simulink model "Lombardy"  (Simulink 7.9)
settings: Solver=ode45  StartTime=0.0  StopTime=10.0  RelTol=1e-3
undefined symbols (not defined in the file or in its folder): f_NODE01, f_NODE02, f_NODE03, f_NODE04, f_NODE05, f_NODE06, f_NODE07, f_NODE08, f_NODE09, f_NODE10, f_NODE11, f_NODE12, f_NODE13, f_NODE14, f_NODE15, f_NODE16, f_NODE17, f_NODE18, f_NODE19, f_NODE20, f_NODE21, f_NODE22, f_NODE23, f_NODE24, f_NODE25, f_NODE26, f_NODE27, f_NODE28, f_NODE29, f_NODE30, f_NODE31, f_NODE32, r_NODE01, r_NODE02, r_NODE03, r_NODE04, r_NODE05, r_NODE06, r_NODE07, r_NODE08, r_NODE09, r_NODE10, r_NODE11, r_NODE12, r_NODE13, r_NODE14, r_NODE15, r_NODE16, r_NODE17, r_NODE18, r_NODE19, r_NODE20, r_NODE21, r_NODE22, r_NODE23, r_NODE24, r_NODE25, r_NODE26, r_NODE27, r_NODE28 ... (+36)
(part 2 of 2)

== system Lombardy/NODE29 ==
  In1 : Inport
  EMF_NODE29 : MATLAB Function  TreatAsAtomicUnit=on
  Gain1_NODE29 : Gain  Gain=-f_NODE29  SaturateOnIntegerOverflow=on  OutDataTypeStr=Inherit: Same as input  ParamDataTypeStr=Inherit: Same as input
  Gain2_NODE29 : Gain  Gain=-r_NODE29  SaturateOnIntegerOverflow=on  OutDataTypeStr=Inherit: Same as input  ParamDataTypeStr=Inherit: Same as input
  Int1_NODE29 : Integrator  InitialCondition=1
  Product1_NODE29 : Product  SaturateOnIntegerOverflow=on  RndMeth=Zero  InputSameDT=on
  ServiceThr1_NODE29 : Constant  Value=th_NODE29
  Set-off1_NODE29 : Constant
  Sum1_NODE29 : Sum  Inputs=|-+  SaturateOnIntegerOverflow=on  InputSameDT=on
  Sum2_NODE29 : Sum  Inputs=|++  SaturateOnIntegerOverflow=on  InputSameDT=on
  Sum3_NODE29 : Sum  Inputs=|+-  SaturateOnIntegerOverflow=on  InputSameDT=on
  WorkSpaceOut_NODE29 : ToWorkspace  VariableName=Out_NODE29
  WorkSpaceState_NODE29 : ToWorkspace  VariableName=State_NODE29
  Out1_NODE29 : Outport
  wires:
  In1/1 -> Gain2_NODE29/1, Sum1_NODE29/1
  Set-off1_NODE29/1 -> Sum1_NODE29/2
  Sum1_NODE29/1 -> Gain1_NODE29/1
  Gain1_NODE29/1 -> Sum2_NODE29/1
  Gain2_NODE29/1 -> Sum2_NODE29/2, Sum3_NODE29/2
  Sum2_NODE29/1 -> Product1_NODE29/1
  Product1_NODE29/1 -> Sum3_NODE29/1
  Int1_NODE29/1 -> Product1_NODE29/2, EMF_NODE29/1(u), WorkSpaceState_NODE29/1
  Sum3_NODE29/1 -> Int1_NODE29/1
  ServiceThr1_NODE29/1 -> EMF_NODE29/2(u0)
  EMF_NODE29/1(y) -> Out1_NODE29/1, WorkSpaceOut_NODE29/1

== system Lombardy/NODE30 ==
  In1 : Inport
  EMF_NODE30 : MATLAB Function  TreatAsAtomicUnit=on
  Gain1_NODE30 : Gain  Gain=-f_NODE30  SaturateOnIntegerOverflow=on  OutDataTypeStr=Inherit: Same as input  ParamDataTypeStr=Inherit: Same as input
  Gain2_NODE30 : Gain  Gain=-r_NODE30  SaturateOnIntegerOverflow=on  OutDataTypeStr=Inherit: Same as input  ParamDataTypeStr=Inherit: Same as input
  Int1_NODE30 : Integrator  InitialCondition=1
  Product1_NODE30 : Product  SaturateOnIntegerOverflow=on  RndMeth=Zero  InputSameDT=on
  ServiceThr1_NODE30 : Constant  Value=th_NODE30
  Set-off1_NODE30 : Constant
  Sum1_NODE30 : Sum  Inputs=|-+  SaturateOnIntegerOverflow=on  InputSameDT=on
  Sum2_NODE30 : Sum  Inputs=|++  SaturateOnIntegerOverflow=on  InputSameDT=on
  Sum3_NODE30 : Sum  Inputs=|+-  SaturateOnIntegerOverflow=on  InputSameDT=on
  WorkSpaceOut_NODE30 : ToWorkspace  VariableName=Out_NODE30
  WorkSpaceState_NODE30 : ToWorkspace  VariableName=State_NODE30
  Out1_NODE30 : Outport
  wires:
  In1/1 -> Gain2_NODE30/1, Sum1_NODE30/1
  Set-off1_NODE30/1 -> Sum1_NODE30/2
  Sum1_NODE30/1 -> Gain1_NODE30/1
  Gain1_NODE30/1 -> Sum2_NODE30/1
  Gain2_NODE30/1 -> Sum2_NODE30/2, Sum3_NODE30/2
  Sum2_NODE30/1 -> Product1_NODE30/1
  Product1_NODE30/1 -> Sum3_NODE30/1
  Int1_NODE30/1 -> Product1_NODE30/2, EMF_NODE30/1(u), WorkSpaceState_NODE30/1
  Sum3_NODE30/1 -> Int1_NODE30/1
  ServiceThr1_NODE30/1 -> EMF_NODE30/2(u0)
  EMF_NODE30/1(y) -> Out1_NODE30/1, WorkSpaceOut_NODE30/1

== system Lombardy/NODE31 ==
  In1 : Inport
  EMF_NODE31 : MATLAB Function  TreatAsAtomicUnit=on
  Gain1_NODE31 : Gain  Gain=-f_NODE31  SaturateOnIntegerOverflow=on  OutDataTypeStr=Inherit: Same as input  ParamDataTypeStr=Inherit: Same as input
  Gain2_NODE31 : Gain  Gain=-r_NODE31  SaturateOnIntegerOverflow=on  OutDataTypeStr=Inherit: Same as input  ParamDataTypeStr=Inherit: Same as input
  Int1_NODE31 : Integrator  InitialCondition=1
  Product1_NODE31 : Product  SaturateOnIntegerOverflow=on  RndMeth=Zero  InputSameDT=on
  ServiceThr1_NODE31 : Constant  Value=th_NODE31
  Set-off1_NODE31 : Constant
  Sum1_NODE31 : Sum  Inputs=|-+  SaturateOnIntegerOverflow=on  InputSameDT=on
  Sum2_NODE31 : Sum  Inputs=|++  SaturateOnIntegerOverflow=on  InputSameDT=on
  Sum3_NODE31 : Sum  Inputs=|+-  SaturateOnIntegerOverflow=on  InputSameDT=on
  WorkSpaceOut_NODE31 : ToWorkspace  VariableName=Out_NODE31
  WorkSpaceState_NODE31 : ToWorkspace  VariableName=State_NODE31
  Out1_NODE31 : Outport
  wires:
  In1/1 -> Gain2_NODE31/1, Sum1_NODE31/1
  Set-off1_NODE31/1 -> Sum1_NODE31/2
  Sum1_NODE31/1 -> Gain1_NODE31/1
  Gain1_NODE31/1 -> Sum2_NODE31/1
  Gain2_NODE31/1 -> Sum2_NODE31/2, Sum3_NODE31/2
  Sum2_NODE31/1 -> Product1_NODE31/1
  Product1_NODE31/1 -> Sum3_NODE31/1
  Int1_NODE31/1 -> Product1_NODE31/2, EMF_NODE31/1(u), WorkSpaceState_NODE31/1
  Sum3_NODE31/1 -> Int1_NODE31/1
  ServiceThr1_NODE31/1 -> EMF_NODE31/2(u0)
  EMF_NODE31/1(y) -> Out1_NODE31/1, WorkSpaceOut_NODE31/1

== system Lombardy/NODE32 ==
  In1 : Inport
  EMF_NODE32 : MATLAB Function  TreatAsAtomicUnit=on
  Gain1_NODE32 : Gain  Gain=-f_NODE32  SaturateOnIntegerOverflow=on  OutDataTypeStr=Inherit: Same as input  ParamDataTypeStr=Inherit: Same as input
  Gain2_NODE32 : Gain  Gain=-r_NODE32  SaturateOnIntegerOverflow=on  OutDataTypeStr=Inherit: Same as input  ParamDataTypeStr=Inherit: Same as input
  Int1_NODE32 : Integrator  InitialCondition=1
  Product1_NODE32 : Product  SaturateOnIntegerOverflow=on  RndMeth=Zero  InputSameDT=on
  ServiceThr1_NODE32 : Constant  Value=th_NODE32
  Set-off1_NODE32 : Constant
  Sum1_NODE32 : Sum  Inputs=|-+  SaturateOnIntegerOverflow=on  InputSameDT=on
  Sum2_NODE32 : Sum  Inputs=|++  SaturateOnIntegerOverflow=on  InputSameDT=on
  Sum3_NODE32 : Sum  Inputs=|+-  SaturateOnIntegerOverflow=on  InputSameDT=on
  WorkSpaceOut_NODE32 : ToWorkspace  VariableName=Out_NODE32
  WorkSpaceState_NODE32 : ToWorkspace  VariableName=State_NODE32
  Out1_NODE32 : Outport
  wires:
  In1/1 -> Gain2_NODE32/1, Sum1_NODE32/1
  Set-off1_NODE32/1 -> Sum1_NODE32/2
  Sum1_NODE32/1 -> Gain1_NODE32/1
  Gain1_NODE32/1 -> Sum2_NODE32/1
  Gain2_NODE32/1 -> Sum2_NODE32/2, Sum3_NODE32/2
  Sum2_NODE32/1 -> Product1_NODE32/1
  Product1_NODE32/1 -> Sum3_NODE32/1
  Int1_NODE32/1 -> Product1_NODE32/2, EMF_NODE32/1(u), WorkSpaceState_NODE32/1
  Sum3_NODE32/1 -> Int1_NODE32/1
  ServiceThr1_NODE32/1 -> EMF_NODE32/2(u0)
  EMF_NODE32/1(y) -> Out1_NODE32/1, WorkSpaceOut_NODE32/1

== matlab function NODE02/EMF_NODE02 ==
  data: u input double; y output double; u0 input double
function y = step(u,  u0)
 if u > u0 
 y=1; 
 else 
 y=0; 
 end

== matlab function NODE01/EMF_NODE01 ==
  data: u input double; y output double; u0 input double
function y = step(u,  u0)
 if u > u0 
 y=1; 
 else 
 y=0; 
 end

== matlab function NODE03/EMF_NODE03 ==
  data: u input double; y output double; u0 input double
function y = step(u,  u0)
 if u > u0 
 y=1; 
 else 
 y=0; 
 end

== matlab function NODE04/EMF_NODE04 ==
  data: u input double; y output double; u0 input double
function y = step(u,  u0)
 if u > u0 
 y=1; 
 else 
 y=0; 
 end

== matlab function NODE05/EMF_NODE05 ==
  data: u input double; y output double; u0 input double
function y = step(u,  u0)
 if u > u0 
 y=1; 
 else 
 y=0; 
 end

== matlab function NODE06/EMF_NODE06 ==
  data: u input double; y output double; u0 input double
function y = step(u,  u0)
 if u > u0 
 y=1; 
 else 
 y=0; 
 end

== matlab function NODE07/EMF_NODE07 ==
  data: u input double; y output double; u0 input double
function y = step(u,  u0)
 if u > u0 
 y=1; 
 else 
 y=0; 
 end

== matlab function NODE08/EMF_NODE08 ==
  data: u input double; y output double; u0 input double
function y = step(u,  u0)
 if u > u0 
 y=1; 
 else 
 y=0; 
 end

== matlab function NODE09/EMF_NODE09 ==
  data: u input double; y output double; u0 input double
function y = step(u,  u0)
 if u > u0 
 y=1; 
 else 
 y=0; 
 end

== matlab function NODE10/EMF_NODE10 ==
  data: u input double; y output double; u0 input double
function y = step(u,  u0)
 if u > u0 
 y=1; 
 else 
 y=0; 
 end

== matlab function NODE11/EMF_NODE11 ==
  data: u input double; y output double; u0 input double
function y = step(u,  u0)
 if u > u0 
 y=1; 
 else 
 y=0; 
 end

== matlab function NODE12/EMF_NODE12 ==
  data: u input double; y output double; u0 input double
function y = step(u,  u0)
 if u > u0 
 y=1; 
 else 
 y=0; 
 end

== matlab function NODE13/EMF_NODE13 ==
  data: u input double; y output double; u0 input double
function y = step(u,  u0)
 if u > u0 
 y=1; 
 else 
 y=0; 
 end

== matlab function NODE14/EMF_NODE14 ==
  data: u input double; y output double; u0 input double
function y = step(u,  u0)
 if u > u0 
 y=1; 
 else 
 y=0; 
 end

== matlab function NODE15/EMF_NODE15 ==
  data: u input double; y output double; u0 input double
function y = step(u,  u0)
 if u > u0 
 y=1; 
 else 
 y=0; 
 end

== matlab function NODE16/EMF_NODE16 ==
  data: u input double; y output double; u0 input double
function y = step(u,  u0)
 if u > u0 
 y=1; 
 else 
 y=0; 
 end

== matlab function NODE17/EMF_NODE17 ==
  data: u input double; y output double; u0 input double
function y = step(u,  u0)
 if u > u0 
 y=1; 
 else 
 y=0; 
 end

== matlab function NODE18/EMF_NODE18 ==
  data: u input double; y output double; u0 input double
function y = step(u,  u0)
 if u > u0 
 y=1; 
 else 
 y=0; 
 end

== matlab function NODE19/EMF_NODE19 ==
  data: u input double; y output double; u0 input double
function y = step(u,  u0)
 if u > u0 
 y=1; 
 else 
 y=0; 
 end

== matlab function NODE20/EMF_NODE20 ==
  data: u input double; y output double; u0 input double
function y = step(u,  u0)
 if u > u0 
 y=1; 
 else 
 y=0; 
 end

== matlab function NODE21/EMF_NODE21 ==
  data: u input double; y output double; u0 input double
function y = step(u,  u0)
 if u > u0 
 y=1; 
 else 
 y=0; 
 end

== matlab function NODE22/EMF_NODE22 ==
  data: u input double; y output double; u0 input double
function y = step(u,  u0)
 if u > u0 
 y=1; 
 else 
 y=0; 
 end

== matlab function NODE23/EMF_NODE23 ==
  data: u input double; y output double; u0 input double
function y = step(u,  u0)
 if u > u0 
 y=1; 
 else 
 y=0; 
 end

== matlab function NODE24/EMF_NODE24 ==
  data: u input double; y output double; u0 input double
function y = step(u,  u0)
 if u > u0 
 y=1; 
 else 
 y=0; 
 end

== matlab function NODE25/EMF_NODE25 ==
  data: u input double; y output double; u0 input double
function y = step(u,  u0)
 if u > u0 
 y=1; 
 else 
 y=0; 
 end

== matlab function NODE26/EMF_NODE26 ==
  data: u input double; y output double; u0 input double
function y = step(u,  u0)
 if u > u0 
 y=1; 
 else 
 y=0; 
 end

== matlab function NODE27/EMF_NODE27 ==
  data: u input double; y output double; u0 input double
function y = step(u,  u0)
 if u > u0 
 y=1; 
 else 
 y=0; 
 end

== matlab function NODE28/EMF_NODE28 ==
  data: u input double; y output double; u0 input double
function y = step(u,  u0)
 if u > u0 
 y=1; 
 else 
 y=0; 
 end

== matlab function NODE29/EMF_NODE29 ==
  data: u input double; y output double; u0 input double
function y = step(u,  u0)
 if u > u0 
 y=1; 
 else 
 y=0; 
 end

== matlab function NODE30/EMF_NODE30 ==
  data: u input double; y output double; u0 input double
function y = step(u,  u0)
 if u > u0 
 y=1; 
 else 
 y=0; 
 end

== matlab function NODE31/EMF_NODE31 ==
  data: u input double; y output double; u0 input double
function y = step(u,  u0)
 if u > u0 
 y=1; 
 else 
 y=0; 
 end

== matlab function NODE32/EMF_NODE32 ==
  data: u input double; y output double; u0 input double
function y = step(u,  u0)
 if u > u0 
 y=1; 
 else 
 y=0; 
 end
